simulink model "Fmacalcul"  (R2019b)
settings: Solver=VariableStepAuto  StartTime=0.0  StopTime=10.0  RelTol=1e-3
values from neighbouring files (symbols this model uses):
  e = 10^-2    (= 0.01)    [run.m]
  n = B0*(zm+e)/(mu*im)    (= 1790.49310978)    [run.m]
  S = p^2    [run.m]
undefined symbols (not defined in the file or in its folder): mu0
settings Model: Creator=anasselhoud  LastModifiedBy=anasselhoud

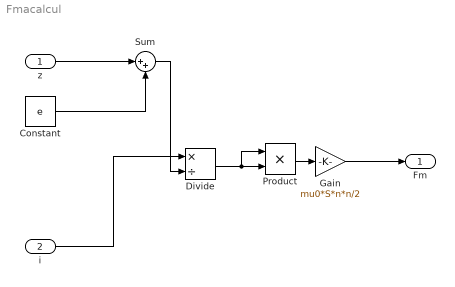
== system Fmacalcul ==
  z : Inport
  i : Inport  Port=2
  Constant : Constant  Value=e
  Divide : Product  Inputs=*/
  Gain : Gain  Gain=mu0*S*n*n/2
  Product : Product
  Sum : Sum  Inputs=|++
  Fm : Outport
  wires:
  Constant/1 -> Sum/2
  z/1 -> Sum/1
  Sum/1 -> Divide/2
  i/1 -> Divide/1
  Divide/1 -> Product/2, Product/1
  Gain/1 -> Fm/1
  Product/1 -> Gain/1
